simulink model "CustArchitecture"  (R2020a)
settings: Solver=FixedStepDiscrete  StartTime=0.0  StopTime=840000  RelTol=1e-3
libraries: IIT_Genoa_Intan_HDL_blocks x7
settings Model: DataTypeOverride=Off  FPTRunName=FPA_Reference  SimulationMode=accelerator  PauseTimes=5600  PacingRate=40  Creator=BuccelliLab  LastModifiedBy=diflo
settings SolverCC: AutoInsertRateTranBlk=on  MinimalZcImpactIntegration=on
settings DataIOCC: LimitDataPoints=on  SaveOutput=off  SaveTime=off  ReturnWorkspaceOutputs=off
settings OptimizationCC: BlockReduction=off  ConditionallyExecuteInputs=off  DefaultParameterBehavior=Inlined  LifeSpan=inf
settings DebuggingCC: SignalRangeChecking=warning  ReadBeforeWriteMsg=DisableAll  WriteAfterWriteMsg=DisableAll  WriteAfterReadMsg=DisableAll  AlgebraicLoopMsg=error  MultiTaskDSMMsg=none  SingleTaskRateTransMsg=error  ParameterDowncastMsg=warning  ParameterOverflowMsg=warning  AllowSymbolicDim=off  StrictBusMsg=ErrorOnBusTreatedAsVector  SFUnexpectedBacktrackingDiag=warning  SFNoUnconditionalDefaultTransitionDiag=warning  SFExecutionAtInitializationDiag=none  ArithmeticOperatorsInVariantConditions=warning
settings HardwareCC: ProdBitPerPointer=32  ProdBitPerSizeT=32  ProdBitPerPtrDiffT=32  ProdLargestAtomicFloat=None  ProdIntDivRoundTo=Undefined  ProdEndianess=Unspecified  ProdWordSize=32  ProdHWDeviceType=ASIC/FPGA->ASIC/FPGA  TargetBitPerPointer=64  TargetBitPerSizeT=64  TargetBitPerPtrDiffT=64  TargetLongLongMode=on  TargetIntDivRoundTo=Zero  TargetEndianess=LittleEndian  TargetWordSize=64  TargetHWDeviceType=Custom Processor->MATLAB Host Computer  ProdEqTarget=off
settings ModelReferenceCC: UpdateModelReferenceTargets=IfOutOfDate
settings SFSimCC: SFSimEcho=off  SimUseLocalCustomCode=off  CustomCodeUndefinedFunction=UseInterfaceOnly
settings RTWCC: RTWUseLocalCustomCode=off
settings CodeAppCC: StateflowObjectComments=on
settings GRTTargetCC: TargetLangStandard=C89/C90 (ANSI)
settings ConfigComp: CovScope=ReferencedModels  CovMetricSettings=dw  CovHtmlReporting=on  CovSaveCumulativeToWorkspaceVar=on  CovSaveSingleToWorkspaceVar=on  CovExternalEMLEnable=off  CovSFcnEnable=off

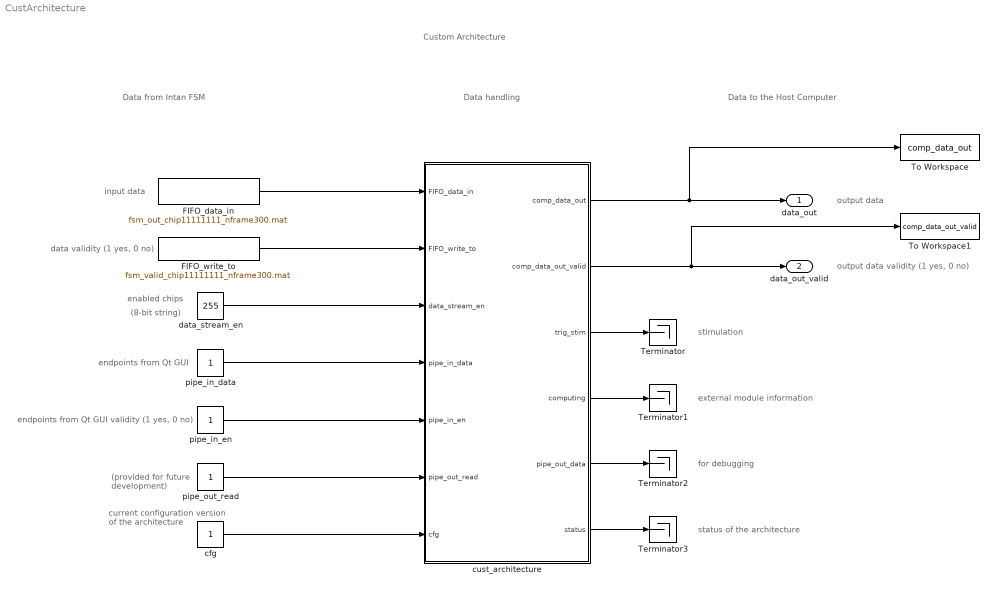
== system CustArchitecture ==
  note: Data handling
  note: Custom Architecture
  note: output data validity (1 yes, 0 no)
  note: endpoints from Qt GUI
  note: (8-bit string)
  note: enabled chips
  note: data validity (1 yes, 0 no)
  note: input data
  note: endpoints from Qt GUI validity (1 yes, 0 no)
  note: (provided for future
      | development)
  note: current configuration
      | version of the
      | architecture
  note: output data
  note: Data to the Host Computer
  note: stimulation
  note: external module information
  note: for debugging
  note: status of the architecture
  note: Data from Intan FSM
  FIFO_data_in : FromFile  FileName=fsm_out_chip11111111_nframe300.mat  OutDataTypeStr=uint16  SampleTime=1  ExtrapolationBeforeFirstDataPoint=Hold first value  InterpolationWithinTimeRange=Zero order hold  ExtrapolationAfterLastDataPoint=Hold last value
  FIFO_write_to : FromFile  FileName=fsm_valid_chip11111111_nframe300.mat  OutDataTypeStr=boolean  SampleTime=1
  Terminator{,1..3} (4 alike) : Terminator
  To Workspace : ToWorkspace  VariableName=comp_data_out  SaveFormat=Timeseries  SampleTime=-1
  To Workspace1 : ToWorkspace  VariableName=comp_data_out_valid  SaveFormat=Timeseries  SampleTime=-1
  cfg : Constant  OutDataTypeStr=uint16  SampleTime=-1
  cust_architecture : Subsystem
  data_stream_en : Constant  Value=255  OutDataTypeStr=uint8  SampleTime=-1
  pipe_in_data : Constant  OutDataTypeStr=uint16  SampleTime=-1
  pipe_in_en : Constant  OutDataTypeStr=boolean  SampleTime=-1
  pipe_out_read : Constant  OutDataTypeStr=boolean  SampleTime=-1
  data_out : Outport  VectorParamsAs1DForOutWhenUnconnected=off
  data_out_valid : Outport  Port=2  VectorParamsAs1DForOutWhenUnconnected=off
  wires:
  FIFO_data_in/1 -> cust_architecture/1(FIFO_data_in)
  FIFO_write_to/1 -> cust_architecture/2(FIFO_write_to)
  cust_architecture/1(comp_data_out) -> To Workspace/1, data_out/1
  cust_architecture/2(comp_data_out_valid) -> To Workspace1/1, data_out_valid/1
  data_stream_en/1 -> cust_architecture/3(data_stream_en)
  pipe_in_data/1 -> cust_architecture/4(pipe_in_data)
  pipe_in_en/1 -> cust_architecture/5(pipe_in_en)
  pipe_out_read/1 -> cust_architecture/6(pipe_out_read)
  cfg/1 -> cust_architecture/7(cfg)
  cust_architecture/3(trig_stim) -> Terminator/1
  cust_architecture/4(computing) -> Terminator1/1
  cust_architecture/5(pipe_out_data) -> Terminator2/1
  cust_architecture/6(status) -> Terminator3/1

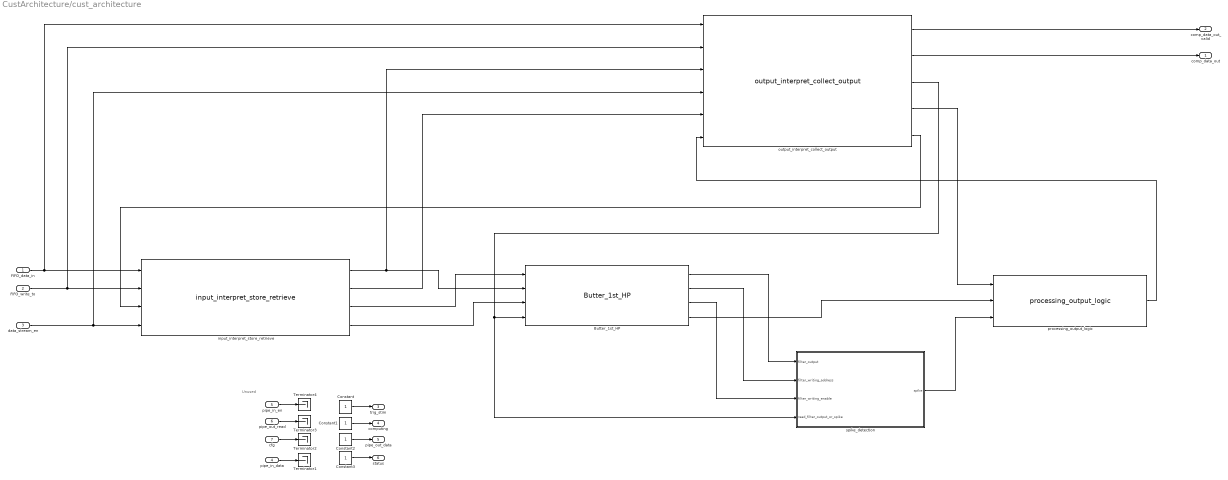
== system CustArchitecture/cust_architecture ==
  note: Unused
  FIFO_data_in : Inport
  FIFO_write_to : Inport  Port=2
  data_stream_en : Inport  Port=3
  pipe_in_data : Inport  Port=4
  pipe_in_en : Inport  Port=5
  pipe_out_read : Inport  Port=6
  cfg : Inport  Port=7
  Butter_1st_HP : IIT_Genoa_Intan_HDL_blocks/Filters/Butter_1st_HP  s1=0.969531252908746199  a21=-0.939062505817492399
      settings: SourceProductName=IIT Genoa Intan HDL blocks
  Constant : Constant  OutDataTypeStr=uint8  SampleTime=-1
  Constant1 : Constant  OutDataTypeStr=boolean  SampleTime=-1
  Constant2 : Constant  OutDataTypeStr=uint16  SampleTime=-1
  Constant3 : Constant  OutDataTypeStr=uint16  SampleTime=-1
  Terminator{1..4} (4 alike) : Terminator
  input_interpret_store_retrieve : IIT_Genoa_Intan_HDL_blocks/Encoding//Decoding/input_interpret_store_retrieve
      settings: SourceProductName=IIT Genoa Intan HDL blocks
  output_interpret_collect_output : IIT_Genoa_Intan_HDL_blocks/Encoding//Decoding/output_interpret_collect_output
      settings: SourceProductName=IIT Genoa Intan HDL blocks
  processing_output_logic : IIT_Genoa_Intan_HDL_blocks/Encoding//Decoding/processing_output_logic
      settings: SourceProductName=IIT Genoa Intan HDL blocks
  spike_detection : Subsystem
  comp_data_out : Outport  VectorParamsAs1DForOutWhenUnconnected=off
  comp_data_out_valid : Outport  Port=2  OutDataTypeStr=boolean  VectorParamsAs1DForOutWhenUnconnected=off
  trig_stim : Outport  Port=3  VectorParamsAs1DForOutWhenUnconnected=off
  computing : Outport  Port=4  VectorParamsAs1DForOutWhenUnconnected=off
  pipe_out_data : Outport  Port=5  VectorParamsAs1DForOutWhenUnconnected=off
  status : Outport  Port=6  VectorParamsAs1DForOutWhenUnconnected=off
  wires:
  Constant/1 -> trig_stim/1
  Constant1/1 -> computing/1
  Constant2/1 -> pipe_out_data/1
  Constant3/1 -> status/1
  cfg/1 -> Terminator2/1
  pipe_out_read/1 -> Terminator3/1
  pipe_in_en/1 -> Terminator4/1
  FIFO_data_in/1 -> input_interpret_store_retrieve/1, output_interpret_collect_output/1
  FIFO_write_to/1 -> input_interpret_store_retrieve/2, output_interpret_collect_output/2
  data_stream_en/1 -> output_interpret_collect_output/4, input_interpret_store_retrieve/4
  pipe_in_data/1 -> Terminator1/1
  output_interpret_collect_output/1 -> comp_data_out_valid/1
  output_interpret_collect_output/2 -> comp_data_out/1
  output_interpret_collect_output/5 -> input_interpret_store_retrieve/3
  output_interpret_collect_output/4 -> processing_output_logic/1
  output_interpret_collect_output/3 -> spike_detection/4(read_filter_output_or_spike), Butter_1st_HP/4
  Butter_1st_HP/4 -> processing_output_logic/2
  input_interpret_store_retrieve/2 -> output_interpret_collect_output/5
  input_interpret_store_retrieve/1 -> Butter_1st_HP/2, output_interpret_collect_output/3
  processing_output_logic/1 -> output_interpret_collect_output/6
  Butter_1st_HP/1 -> spike_detection/1(filter_output)
  Butter_1st_HP/2 -> spike_detection/2(filter_writing_address)
  Butter_1st_HP/3 -> spike_detection/3(filter_writing_enable)
  spike_detection/1(spike) -> processing_output_logic/3
  input_interpret_store_retrieve/3 -> Butter_1st_HP/1
  input_interpret_store_retrieve/4 -> Butter_1st_HP/3

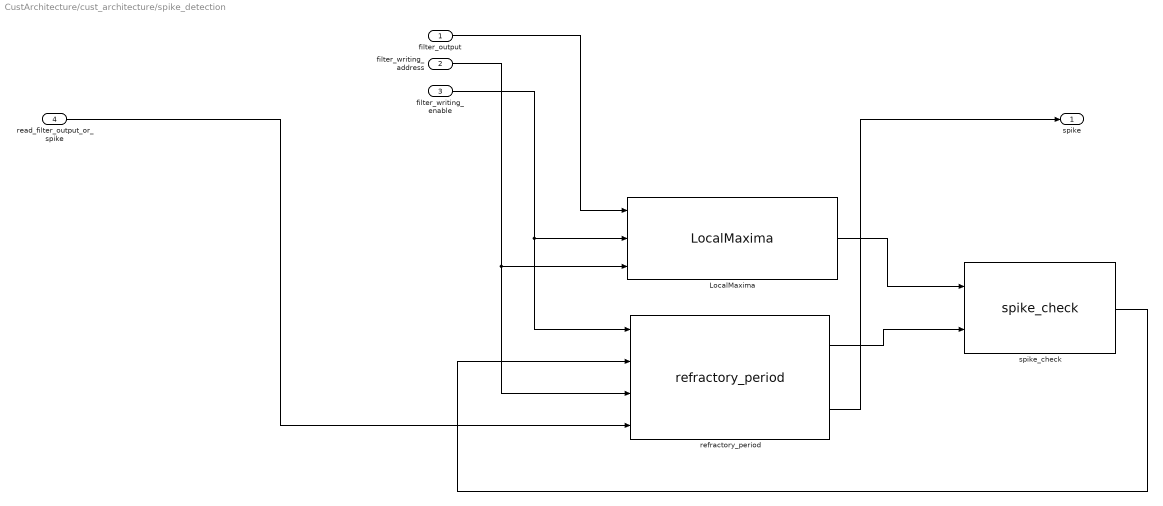
== system CustArchitecture/cust_architecture/spike_detection ==
  filter_output : Inport
  filter_writing_address : Inport  Port=2
  filter_writing_enable : Inport  Port=3
  read_filter_output_or_spike : Inport  Port=4
  LocalMaxima : IIT_Genoa_Intan_HDL_blocks/Spike Detection/Sample Thresholding/LocalMaxima  th=0
      settings: SourceProductName=IIT Genoa Intan HDL blocks
  refractory_period : IIT_Genoa_Intan_HDL_blocks/Spike Detection/General/refractory_period  refractory=30
      settings: SourceProductName=IIT Genoa Intan HDL blocks
  spike_check : IIT_Genoa_Intan_HDL_blocks/Spike Detection/General/spike_check
      settings: SourceProductName=IIT Genoa Intan HDL blocks
  spike : Outport
  wires:
  spike_check/1 -> refractory_period/2
  LocalMaxima/1 -> spike_check/1
  filter_writing_address/1 -> refractory_period/3, LocalMaxima/3
  refractory_period/1 -> spike_check/2
  filter_writing_enable/1 -> refractory_period/1, LocalMaxima/2
  filter_output/1 -> LocalMaxima/1
  read_filter_output_or_spike/1 -> refractory_period/4
  refractory_period/2 -> spike/1
